simulink model "ManulControlAPI"  (R2020b)
settings: Solver=ode4  StartTime=0.0  StopTime=inf  FixedStep=0.01  RelTol=1e-3
libraries: etargetslib x2, sharedtransform x1, slrealtimeiplib x1
settings Model: EnablePacing=on  Creator=dream  LastModifiedBy=kcx06
settings DebuggingCC: ArithmeticOperatorsInVariantConditions=warning
settings SFSimCC: SimUseLocalCustomCode=off  CustomCodeUndefinedFunction=UseInterfaceOnly
settings RTWCC: RTWUseLocalCustomCode=off

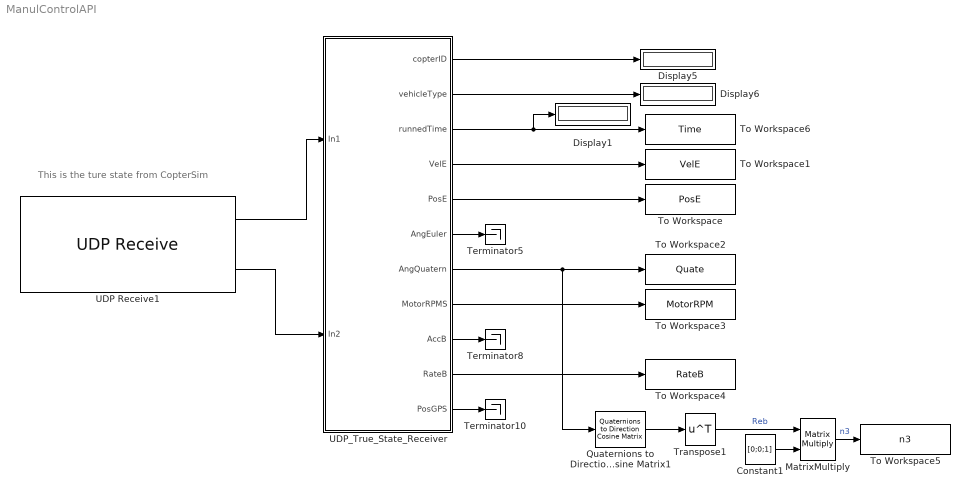
== system ManulControlAPI ==
  note: This is the ture state from CopterSim
  Constant1 : Constant  Value=[0;0;1]
  Display1 : Display
  Display5 : Display
  Display6 : Display
  MatrixMultiply : Product  Multiplication=Matrix(*)
  Quaternions to Direction Cosine Matrix1 : sharedtransform/Quaternions to  Direction Cosine Matrix  aMode=aMode
      settings: SourceProductBaseCode=AE,PW,MT,UV,VE,VP
  Terminator10 : Terminator
  Terminator5 : Terminator
  Terminator8 : Terminator
  To Workspace : ToWorkspace  VariableName=PosE  SaveFormat=Timeseries  SampleTime=-1
  To Workspace1 : ToWorkspace  VariableName=VelE  SaveFormat=Timeseries  SampleTime=-1
  To Workspace2 : ToWorkspace  VariableName=Quate  SaveFormat=Timeseries  SampleTime=-1
  To Workspace3 : ToWorkspace  VariableName=MotorRPM  SaveFormat=Timeseries  SampleTime=-1
  To Workspace4 : ToWorkspace  VariableName=RateB  SaveFormat=Timeseries  SampleTime=-1
  To Workspace5 : ToWorkspace  VariableName=n3  SaveFormat=Timeseries  SampleTime=-1
  To Workspace6 : ToWorkspace  VariableName=Time  SaveFormat=Timeseries  SampleTime=-1
  Transpose1 : Math  Operator=transpose  SaturateOnIntegerOverflow=on
  UDP Receive1 : slrealtimeiplib/UDP Receive  useHostTargetConn=on  ipAddress=10.10.10.15  localPort=20010  rcvWidth=200  rcvFmAny=on  fmAddress=0.0.0.0  rcvMulticast=off  multicastAddress={}  sampleTime=-1
      settings: SourceProductBaseCode=XP
  UDP_True_State_Receiver : Subsystem
  wires:
  UDP_True_State_Receiver/6(AngEuler) -> Terminator5/1
  UDP_True_State_Receiver/8(MotorRPMS) -> To Workspace3/1
  UDP_True_State_Receiver/11(PosGPS) -> Terminator10/1
  UDP_True_State_Receiver/9(AccB) -> Terminator8/1
  UDP_True_State_Receiver/2(vehicleType) -> Display6/1
  UDP_True_State_Receiver/7(AngQuatern) -> To Workspace2/1, Quaternions to Direction Cosine Matrix1/1
  UDP_True_State_Receiver/10(RateB) -> To Workspace4/1
  UDP_True_State_Receiver/4(VelE) -> To Workspace1/1
  UDP Receive1/2 -> UDP_True_State_Receiver/2(In2)
  UDP_True_State_Receiver/1(copterID) -> Display5/1
  UDP_True_State_Receiver/5(PosE) -> To Workspace/1
  UDP_True_State_Receiver/3(runnedTime) -> Display1/1, To Workspace6/1
  UDP Receive1/1 -> UDP_True_State_Receiver/1(In1)
  Constant1/1 -> MatrixMultiply/2
  Quaternions to Direction Cosine Matrix1/1 -> Transpose1/1
  MatrixMultiply/1 -> To Workspace5/1  "n3"
  Transpose1/1 -> MatrixMultiply/1  "Reb"

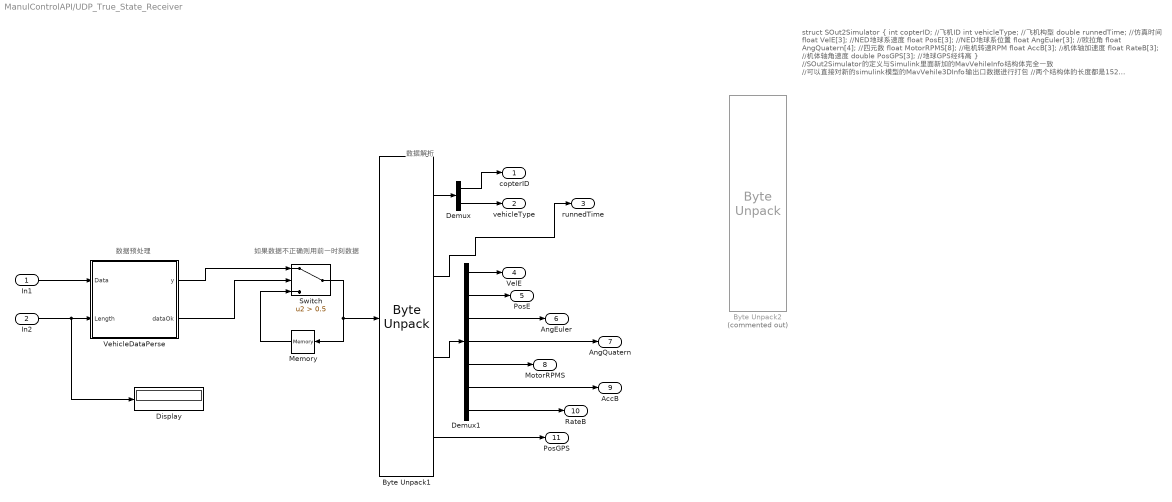
== system ManulControlAPI/UDP_True_State_Receiver ==
  note: 数据解析
  note: 数据预处理
  note: 如果数据不正确则用前一时刻数据
  note: struct SOut2Simulator
      | {
      | int copterID; //飞机ID
      | int vehicleType; //飞机构型
      | double runnedTime; //仿真时间
      | float VelE[3]; //NED地球系速度
      | float PosE[3]; //NED地球系位置
      | float AngEuler[3]; //欧拉角
      | float AngQuatern[4]; //四元数
      | float MotorRPMS[8]; //电机转速RPM
      | float AccB[3]; //机体轴加速度
      | float RateB[3]; //机体轴角速度
      | double PosGPS[3]; //地球GPS经纬高
      | }
      |
      | //SOut2Simulator的定义与Simulink里面新加的MavVehileInfo结构体完全一致
      | //可以直接对新的simulink模型的MavVehile3DInfo输出口数据进行打包
      | //两个结构体的长度都是152
      | sizeof(SOut2Simulator) = sizeof(MavVehileInfo) = 152
      |
      | 打包封装的结构体为
      | typedef struct _netDataShort
      | {
      | TargetType tg; //这里目前随便填，写1即可 uint32
      | int len; //这个长度为传输结构体长度，目前是152
      | char payload[192]; //这里面前152位存放了SOut2Simulator结构体数据，后面的40位保留
      | }netDataShort;
      |
      | //UDP包的总长度为200
      | sizeof(netDataShort) = 200
      |
      | //发送的UDP端口号为：20010
  In1 : Inport
  In2 : Inport  Port=2
  Byte Unpack1 : etargetslib/Byte Unpack  dimensions={2,1,27,3}  datatypes={'int32','double','single','double'}  byteAlign=8
  Byte Unpack2 : etargetslib/Byte Unpack  Commented=on  dimensions={1,1,1,3,3,3,4,8,3,3,3}  datatypes={'int32','int32','double','single','single','single','single','single','single','single','double'}  byteAlign=1
  Demux : Demux  Outputs=2
  Demux1 : Demux  Outputs=[3,3,3,4,8,3,3]
  Display : Display
  Memory : Memory  InitialCondition=uint8(zeros(152,1))
  Switch : Switch  Criteria=u2 > Threshold  Threshold=0.5
  VehicleDataPerse : MATLAB Function  TreatAsAtomicUnit=on
  copterID : Outport  VectorParamsAs1DForOutWhenUnconnected=off
  vehicleType : Outport  Port=2  VectorParamsAs1DForOutWhenUnconnected=off
  runnedTime : Outport  Port=3  VectorParamsAs1DForOutWhenUnconnected=off
  VelE : Outport  Port=4  VectorParamsAs1DForOutWhenUnconnected=off
  PosE : Outport  Port=5  VectorParamsAs1DForOutWhenUnconnected=off
  AngEuler : Outport  Port=6  VectorParamsAs1DForOutWhenUnconnected=off
  AngQuatern : Outport  Port=7  VectorParamsAs1DForOutWhenUnconnected=off
  MotorRPMS : Outport  Port=8  VectorParamsAs1DForOutWhenUnconnected=off
  AccB : Outport  Port=9  VectorParamsAs1DForOutWhenUnconnected=off
  RateB : Outport  Port=10  VectorParamsAs1DForOutWhenUnconnected=off
  PosGPS : Outport  Port=11  VectorParamsAs1DForOutWhenUnconnected=off
  wires:
  VehicleDataPerse/2(dataOk) -> Switch/2
  In2/1 -> Display/1, VehicleDataPerse/2(Length)
  In1/1 -> VehicleDataPerse/1(Data)
  VehicleDataPerse/1(y) -> Switch/1
  Switch/1 -> Memory/1, Byte Unpack1/1
  Memory/1 -> Switch/3
  Byte Unpack1/1 -> Demux/1
  Demux/1 -> copterID/1
  Demux/2 -> vehicleType/1
  Byte Unpack1/2 -> runnedTime/1
  Byte Unpack1/3 -> Demux1/1
  Demux1/1 -> VelE/1
  Demux1/2 -> PosE/1
  Demux1/3 -> AngEuler/1
  Demux1/4 -> AngQuatern/1
  Demux1/5 -> MotorRPMS/1
  Demux1/6 -> AccB/1
  Demux1/7 -> RateB/1
  Byte Unpack1/4 -> PosGPS/1

== matlab function ManulControlAPI/UDP_True_State_Receiver/VehicleDataPerse ==
  data: Data input; y output uint8 size=[152,1]; Length input; dataOk output
function [y,dataOk] = fcn(Data,Length)
y=uint8(zeros(152,1));
dataOk = 0;
if Length ~= 200
    return;
end
len = typecast(Data(5:8), 'int32');

if len ~= 152
   return; 
end

y = Data(9:160);
dataOk = 1;
